simulink model "HighClearance_model"  (R2019b)
settings: configuration reference "configRef" (kept outside this file)
undefined symbols (not defined in the file): baseClearance, calSTEP1_e, calSTEP2_e, calSTEP3_e, calSTEP4_e, calTolMultiplier, errorMinSpd, heightCalibrating_e, heightDiffTolerance, heightDown_e, heightError_e, heightMovingDown_e, heightMovingUp_e, heightUnknown_e, heightUp_e, IOD_OK, IOD_Open, IOD_ScGnd, maxMedianWheelAngle, maxTransitionMachineSpd, minTransitionMachineSpd, positionSensor_tblData, positionSensorFL_BrkPnts, positionSensorFR_BrkPnts, positionSensorRL_BrkPnts, positionSensorRR_BrkPnts, step_time, trackWidthMax, trackWidthMin, trackWidthTolerance, twoWheelSteer
libraries: HighClearance_library x129, simulink x25
(part 1 of 3)
settings Model: Creator=lemaya  LastModifiedBy=lemaya
settings ConfigSetRef: SourceName=configRef  SourceLocation=Base Workspace

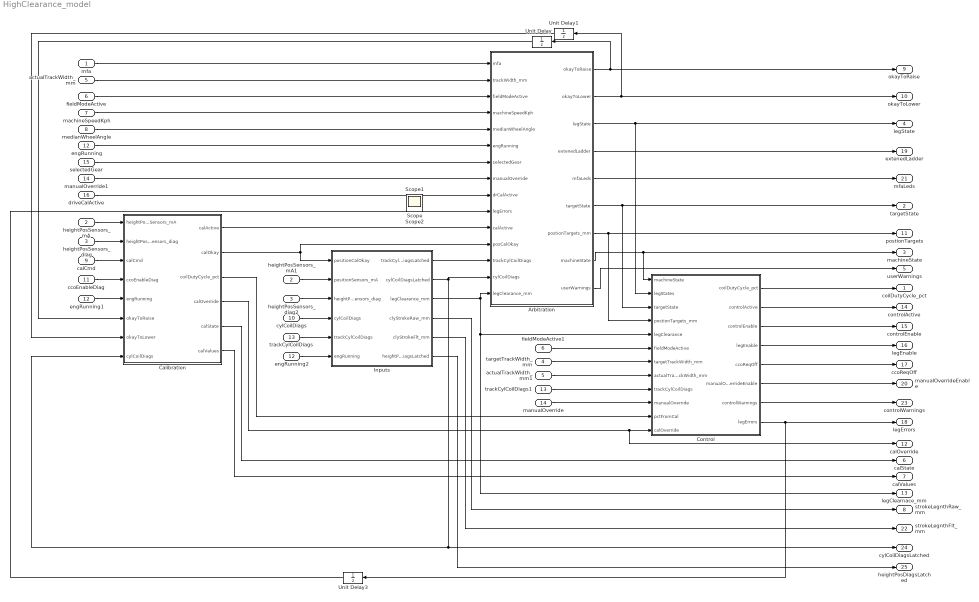
== system HighClearance_model ==
  mfa : Inport  OutDataTypeStr=Bus: MfaBus
  heightPosSensors_mA : Inport  Port=2  OutDataTypeStr=Bus: CylinderBus
  heightPosSensors_diag : Inport  Port=3  OutDataTypeStr=Bus: StateBus
  targetTrackWidth_mm : Inport  Port=4  OutDataTypeStr=Bus: CylinderBus
  actualTrackWidth_mm : Inport  Port=5  OutDataTypeStr=Bus: CylinderBus
  fieldModeActive : Inport  Port=6
  machineSpeedKph : Inport  Port=7
  medianWheelAngle : Inport  Port=8
  calCmd : Inport  Port=9
  cylCoilDiags : Inport  Port=10  OutDataTypeStr=Bus: CoilStateBus
  ccoEnableDiag : Inport  Port=11  OutDataTypeStr=uint8
  engRunning : Inport  Port=12  OutDataTypeStr=boolean
  trackCylCoilDiags : Inport  Port=13  OutDataTypeStr=Bus: CoilStateBus
  manualOverride : Inport  Port=14
  selectedGear : Inport  Port=15
  driveCalActive : Inport  Port=16
  Arbitration : Subsystem
  Calibration : Subsystem
  Control : Subsystem
  Inputs : Subsystem
  Unit Delay : UnitDelay  SampleTime=-1  HasFrameUpgradeWarning=on
  Unit Delay1 : UnitDelay  SampleTime=-1  HasFrameUpgradeWarning=on
  Unit Delay3 : UnitDelay  SampleTime=-1  HasFrameUpgradeWarning=on
  actualTrackWidth_mm1 : InportShadow  Port=5  OutDataTypeStr=Bus: CylinderBus
  engRunning1 : InportShadow  Port=12  OutDataTypeStr=boolean
  engRunning2 : InportShadow  Port=12  OutDataTypeStr=boolean
  fieldModeActive1 : InportShadow  Port=6
  heightPosSensors_diag2 : InportShadow  Port=3  OutDataTypeStr=Bus: StateBus
  heightPosSensors_mA1 : InportShadow  Port=2  OutDataTypeStr=Bus: CylinderBus
  manualOverride1 : InportShadow  Port=14
  trackCylCoilDiags1 : InportShadow  Port=13  OutDataTypeStr=Bus: CoilStateBus
  coilDutyCycle_pct : Outport  OutDataTypeStr=Bus: CoilBus
  targetState : Outport  Port=2
  machineState : Outport  Port=3
  legState : Outport  Port=4  OutDataTypeStr=Bus: StateBus
  userWarnings : Outport  Port=5  OutDataTypeStr=Bus: UserWarningBus
  calState : Outport  Port=6
  calValues : Outport  Port=7  OutDataTypeStr=Bus: CoilBus
  strokeLegnthRaw_mm : Outport  Port=8  OutDataTypeStr=Bus: CylinderBus
  okayToRaise : Outport  Port=9
  okayToLower : Outport  Port=10
  postionTargets : Outport  Port=11  OutDataTypeStr=Bus: CylinderBus
  calOverride : Outport  Port=12
  legClearnace_mm : Outport  Port=13  OutDataTypeStr=Bus: CylinderBus
  controlActive : Outport  Port=14
  controlEnable : Outport  Port=15
  legEnable : Outport  Port=16  OutDataTypeStr=Bus: StateBus
  ccoReqOff : Outport  Port=17
  legErrors : Outport  Port=18  OutDataTypeStr=Bus: ErrorsBus
  extenedLadder : Outport  Port=19
  manualOverrideEnable : Outport  Port=20
  mfaLeds : Outport  Port=21  OutDataTypeStr=Bus: MfaBus
  strokeLegnthFlt_mm : Outport  Port=22  OutDataTypeStr=Bus: CylinderBus
  controlWarnings : Outport  Port=23  OutDataTypeStr=Bus: ControlWarningsBus  BusOutputAsStruct=on
  cylCoilDiagsLatched : Outport  Port=24  OutDataTypeStr=Bus: CoilStateBus
  heightPosDiagsLatched : Outport  Port=25  OutDataTypeStr=Bus: StateBus
  Scope : Scope
  Scope1 : Scope
  Scope2 : Scope
  wires:
  heightPosSensors_mA1/1 -> Inputs/2(positionSensors_mA)
  Inputs/4(clyStrokeRaw_mm) -> strokeLegnthRaw_mm/1
  actualTrackWidth_mm/1 -> Arbitration/2(trackWidth_mm)
  mfa/1 -> Arbitration/1(mfa)
  Arbitration/7(postionTargets_mm) -> Control/4(postionTargets_mm), postionTargets/1
  actualTrackWidth_mm1/1 -> Control/8(actualTrackWidth_mm)
  Arbitration/6(targetState) -> Control/3(targetState), targetState/1
  Arbitration/8(machineState) -> Control/1(machineState), machineState/1
  Arbitration/3(legState) -> Control/2(legStates), legState/1
  fieldModeActive/1 -> Arbitration/3(fieldModeActive)
  targetTrackWidth_mm/1 -> Control/7(targetTrackWidth_mm)
  Arbitration/9(userWarnings) -> userWarnings/1
  machineSpeedKph/1 -> Arbitration/4(machineSpeedKph)
  medianWheelAngle/1 -> Arbitration/5(medianWheelAngle)
  Calibration/1(calActive) -> Arbitration/11(calActive)
  Calibration/2(calOkay) -> Inputs/1(positionCalOkay), Arbitration/12(posCalOkay)
  heightPosSensors_mA/1 -> Calibration/1(heightPosSensors_mA)
  heightPosSensors_diag/1 -> Calibration/2(heightPosSensors_diag)
  calCmd/1 -> Calibration/3(calCmd)
  Calibration/5(calState) -> calState/1
  Calibration/3(coilDutyCycle_pct) -> Control/11(pctFromCal)
  Calibration/4(calOverride) -> Control/12(calOverride), calOverride/1
  Calibration/6(calValues) -> calValues/1
  ccoEnableDiag/1 -> Calibration/4(ccoEnableDiag)
  engRunning/1 -> Arbitration/6(engRunning)
  Arbitration/1(okayToRaise) -> Unit Delay/1, okayToRaise/1
  Arbitration/2(okayToLower) -> Unit Delay1/1, okayToLower/1
  Unit Delay/1 -> Calibration/6(okayToRaise)
  Unit Delay1/1 -> Calibration/7(okayToLower)
  Control/1(coilDutyCycle_pct) -> coilDutyCycle_pct/1
  heightPosSensors_diag2/1 -> Inputs/3(heightPosSensors_diag)
  Inputs/3(legClearance_mm) -> Arbitration/15(legClearance_mm), legClearnace_mm/1, Control/5(legClearance)
  Control/2(controlActive) -> controlActive/1
  Control/3(controlEnable) -> controlEnable/1
  Control/4(legEnable) -> legEnable/1
  Control/5(ccoReqOff) -> ccoReqOff/1
  Control/8(legErrors) -> legErrors/1, Unit Delay3/1
  Unit Delay3/1 -> Arbitration/10(legErrors)
  manualOverride/1 -> Control/10(manualOverride)
  selectedGear/1 -> Arbitration/7(selectedGear)
  Arbitration/4(extenedLadder) -> extenedLadder/1
  Control/6(manualOverrideEnable) -> manualOverrideEnable/1
  Arbitration/5(mfaLeds) -> mfaLeds/1
  Inputs/5(clyStrokeFlt_mm) -> strokeLegnthFlt_mm/1
  manualOverride1/1 -> Arbitration/8(manualOverride)
  Control/7(controlWarnings) -> controlWarnings/1
  driveCalActive/1 -> Arbitration/9(drCalActive)
  cylCoilDiags/1 -> Inputs/4(cylCoilDiags)
  Inputs/2(cylCoilDiagsLatched) -> Arbitration/14(cylCoilDiags), Calibration/8(cylCoilDiags), cylCoilDiagsLatched/1
  Inputs/1(trackCylCoilDiagsLatched) -> Arbitration/13(trackCylCoilDiags)
  trackCylCoilDiags/1 -> Inputs/5(trackCylCoilDiags)
  trackCylCoilDiags1/1 -> Control/9(trackCylCoilDiags)
  engRunning1/1 -> Calibration/5(engRunning)
  fieldModeActive1/1 -> Control/6(fieldModeActive)
  Inputs/6(heightPosDiagsLatched) -> heightPosDiagsLatched/1
  engRunning2/1 -> Inputs/6(engRunning)

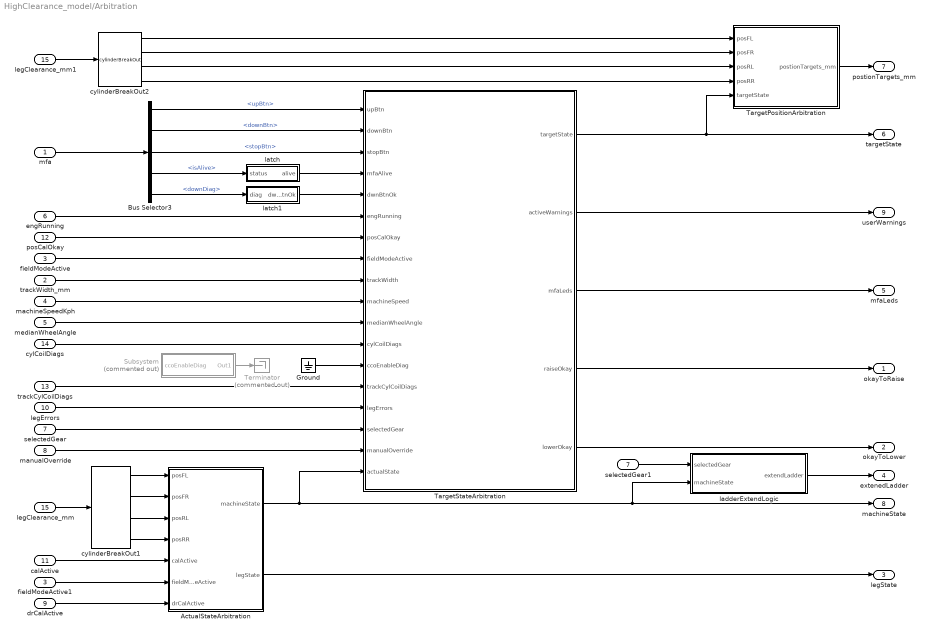
== system HighClearance_model/Arbitration ==
  mfa : Inport  OutDataTypeStr=Bus: MfaBus
  trackWidth_mm : Inport  Port=2  OutDataTypeStr=Bus: CylinderBus
  fieldModeActive : Inport  Port=3
  machineSpeedKph : Inport  Port=4
  medianWheelAngle : Inport  Port=5
  engRunning : Inport  Port=6
  selectedGear : Inport  Port=7
  manualOverride : Inport  Port=8
  drCalActive : Inport  Port=9
  legErrors : Inport  Port=10  OutDataTypeStr=Bus: ErrorsBus
  calActive : Inport  Port=11
  posCalOkay : Inport  Port=12
  trackCylCoilDiags : Inport  Port=13  OutDataTypeStr=Bus: CoilStateBus
  cylCoilDiags : Inport  Port=14  OutDataTypeStr=Bus: CoilStateBus
  legClearance_mm : Inport  Port=15  OutDataTypeStr=Bus: CylinderBus
  ActualStateArbitration : Subsystem
  Bus Selector3 : BusSelector  OutputSignals=upBtn,downBtn,stopBtn,isAlive,downDiag
  Ground : Ground
  Subsystem : Subsystem  Commented=on
  TargetPositionArbitration : Subsystem
  TargetStateArbitration : Stateflow chart  TreatAsAtomicUnit=on
  Terminator : Terminator  Commented=on
  cylinderBreakOut1 : HighClearance_library/cylinderBreakOut  SystemSampleTime=-1  Latency=0  AutoFrameSizeCalculation=off
  cylinderBreakOut2 : HighClearance_library/cylinderBreakOut  SystemSampleTime=-1  Latency=0  AutoFrameSizeCalculation=off
  fieldModeActive1 : InportShadow  Port=3
  ladderExtendLogic : Stateflow chart  TreatAsAtomicUnit=on
      settings: AttributesFormatString=%<Description> Note: Ladder extention not used
  latch : Stateflow chart  TreatAsAtomicUnit=on
  latch1 : Stateflow chart  TreatAsAtomicUnit=on
  legClearance_mm1 : InportShadow  Port=15  OutDataTypeStr=Bus: CylinderBus
  selectedGear1 : InportShadow  Port=7
  okayToRaise : Outport
  okayToLower : Outport  Port=2
  legState : Outport  Port=3  OutDataTypeStr=Bus: StateBus
  extenedLadder : Outport  Port=4
  mfaLeds : Outport  Port=5  OutDataTypeStr=Bus: MfaBus
  targetState : Outport  Port=6
  postionTargets_mm : Outport  Port=7  OutDataTypeStr=Bus: CylinderBus
  machineState : Outport  Port=8
  userWarnings : Outport  Port=9  OutDataTypeStr=Bus: UserWarningBus
  wires:
  ActualStateArbitration/2(legState) -> legState/1
  ActualStateArbitration/1(machineState) -> TargetStateArbitration/18(actualState), ladderExtendLogic/2(machineState), machineState/1
  TargetStateArbitration/1(targetState) -> targetState/1, TargetPositionArbitration/5(targetState)
  TargetPositionArbitration/1(postionTargets_mm) -> postionTargets_mm/1
  mfa/1 -> Bus Selector3/1
  Bus Selector3/2 -> TargetStateArbitration/2(downBtn)  "<downBtn>"
  Bus Selector3/1 -> TargetStateArbitration/1(upBtn)  "<upBtn>"
  Bus Selector3/3 -> TargetStateArbitration/3(stopBtn)  "<stopBtn>"
  TargetStateArbitration/2(activeWarnings) -> userWarnings/1
  calActive/1 -> ActualStateArbitration/5(calActive)
  cylinderBreakOut1/4 -> ActualStateArbitration/4(posRR)
  cylinderBreakOut1/3 -> ActualStateArbitration/3(posRL)
  cylinderBreakOut1/2 -> ActualStateArbitration/2(posFR)
  cylinderBreakOut1/1 -> ActualStateArbitration/1(posFL)
  legClearance_mm/1 -> cylinderBreakOut1/1
  legClearance_mm1/1 -> cylinderBreakOut2/1
  cylinderBreakOut2/1 -> TargetPositionArbitration/1(posFL)
  cylinderBreakOut2/2 -> TargetPositionArbitration/2(posFR)
  cylinderBreakOut2/3 -> TargetPositionArbitration/3(posRL)
  cylinderBreakOut2/4 -> TargetPositionArbitration/4(posRR)
  trackWidth_mm/1 -> TargetStateArbitration/9(trackWidth)
  fieldModeActive/1 -> TargetStateArbitration/8(fieldModeActive)
  machineSpeedKph/1 -> TargetStateArbitration/10(machineSpeed)
  medianWheelAngle/1 -> TargetStateArbitration/11(medianWheelAngle)
  cylCoilDiags/1 -> TargetStateArbitration/12(cylCoilDiags)
  posCalOkay/1 -> TargetStateArbitration/7(posCalOkay)
  engRunning/1 -> TargetStateArbitration/6(engRunning)
  trackCylCoilDiags/1 -> TargetStateArbitration/14(trackCylCoilDiags)
  TargetStateArbitration/4(raiseOkay) -> okayToRaise/1
  TargetStateArbitration/5(lowerOkay) -> okayToLower/1
  legErrors/1 -> TargetStateArbitration/15(legErrors)
  selectedGear/1 -> TargetStateArbitration/16(selectedGear)
  selectedGear1/1 -> ladderExtendLogic/1(selectedGear)
  ladderExtendLogic/1(extendLadder) -> extenedLadder/1
  TargetStateArbitration/3(mfaLeds) -> mfaLeds/1
  manualOverride/1 -> TargetStateArbitration/17(manualOverride)
  Subsystem/1(Out1) -> Terminator/1
  Ground/1 -> TargetStateArbitration/13(ccoEnableDiag)
  Bus Selector3/4 -> latch/1(status)  "<isAlive>"
  latch/1(alive) -> TargetStateArbitration/4(mfaAlive)
  fieldModeActive1/1 -> ActualStateArbitration/6(fieldModeActive)
  drCalActive/1 -> ActualStateArbitration/7(drCalActive)
  Bus Selector3/5 -> latch1/1(diag)  "<downDiag>"
  latch1/1(dwnBtnOk) -> TargetStateArbitration/5(dwnBtnOk)

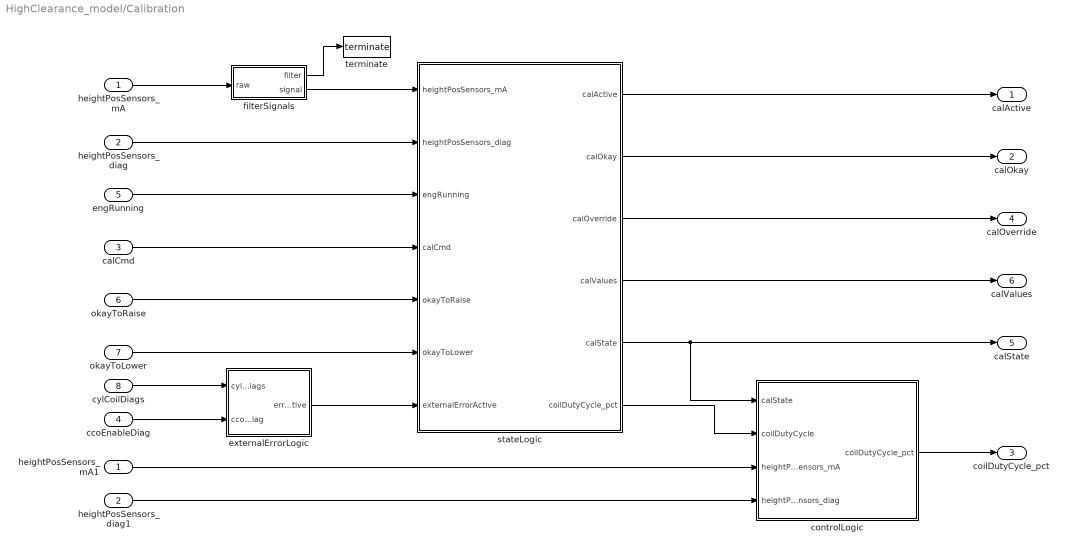
== system HighClearance_model/Calibration ==
  heightPosSensors_mA : Inport  OutDataTypeStr=Bus: CylinderBus
  heightPosSensors_diag : Inport  Port=2  OutDataTypeStr=Bus: StateBus
  calCmd : Inport  Port=3
  ccoEnableDiag : Inport  Port=4
  engRunning : Inport  Port=5  OutDataTypeStr=boolean
  okayToRaise : Inport  Port=6
  okayToLower : Inport  Port=7
  cylCoilDiags : Inport  Port=8  OutDataTypeStr=Bus: CoilStateBus
  controlLogic : Subsystem
  externalErrorLogic : Subsystem
  filterSignals : Subsystem
  heightPosSensors_diag1 : InportShadow  Port=2  OutDataTypeStr=Bus: StateBus
  heightPosSensors_mA1 : InportShadow  OutDataTypeStr=Bus: CylinderBus
  stateLogic : Subsystem
  terminate : HighClearance_library/terminate  SystemSampleTime=-1  Latency=0  AutoFrameSizeCalculation=off
  calActive : Outport
  calOkay : Outport  Port=2
  coilDutyCycle_pct : Outport  Port=3  OutDataTypeStr=Bus: CoilBus
  calOverride : Outport  Port=4
  calState : Outport  Port=5
  calValues : Outport  Port=6
  wires:
  heightPosSensors_mA/1 -> filterSignals/1(raw)
  heightPosSensors_diag/1 -> stateLogic/2(heightPosSensors_diag)
  calCmd/1 -> stateLogic/4(calCmd)
  stateLogic/1(calActive) -> calActive/1
  stateLogic/2(calOkay) -> calOkay/1
  stateLogic/5(calState) -> controlLogic/1(calState), calState/1
  stateLogic/3(calOverride) -> calOverride/1
  stateLogic/6(coilDutyCycle_pct) -> controlLogic/2(coilDutyCycle)
  heightPosSensors_mA1/1 -> controlLogic/3(heightPosSensors_mA)
  controlLogic/1(coilDutyCycle_pct) -> coilDutyCycle_pct/1
  stateLogic/4(calValues) -> calValues/1
  ccoEnableDiag/1 -> externalErrorLogic/2(ccoEnableDiag)
  cylCoilDiags/1 -> externalErrorLogic/1(cylCoilDiags)
  externalErrorLogic/1(errorActive) -> stateLogic/7(externalErrorActive)
  okayToRaise/1 -> stateLogic/5(okayToRaise)
  okayToLower/1 -> stateLogic/6(okayToLower)
  heightPosSensors_diag1/1 -> controlLogic/4(heightPosSensors_diag)
  filterSignals/1(filter) -> terminate/1
  filterSignals/2(signal) -> stateLogic/1(heightPosSensors_mA)
  engRunning/1 -> stateLogic/3(engRunning)

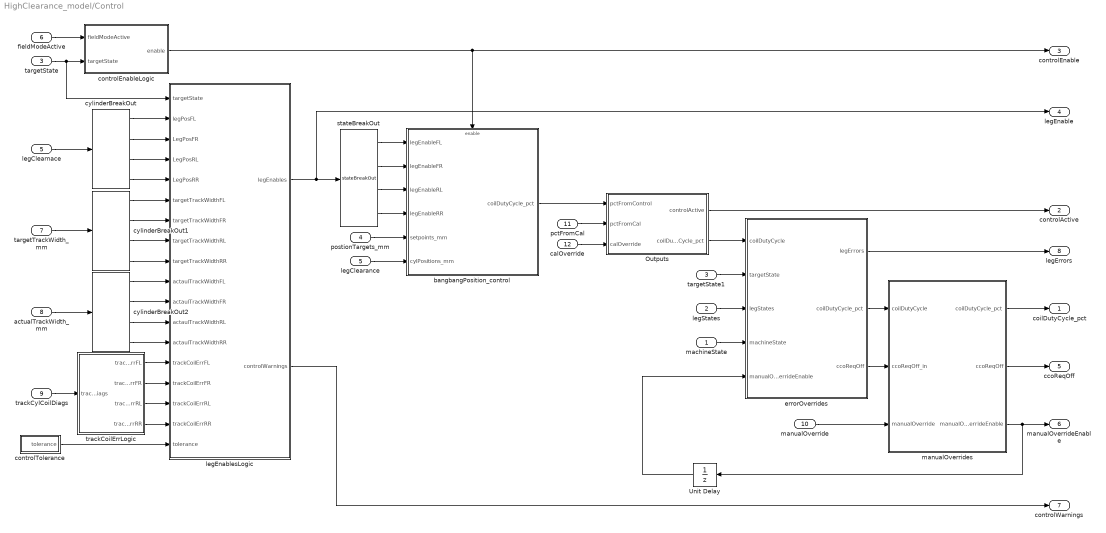
== system HighClearance_model/Control ==
  machineState : Inport
  legStates : Inport  Port=2  OutDataTypeStr=Bus: StateBus
  targetState : Inport  Port=3
  postionTargets_mm : Inport  Port=4  OutDataTypeStr=Bus: CylinderBus
  legClearance : Inport  Port=5  OutDataTypeStr=Bus: CylinderBus
  fieldModeActive : Inport  Port=6
  targetTrackWidth_mm : Inport  Port=7  OutDataTypeStr=Bus: CylinderBus
  actualTrackWidth_mm : Inport  Port=8  OutDataTypeStr=Bus: CylinderBus
  trackCylCoilDiags : Inport  Port=9  OutDataTypeStr=Bus: CoilStateBus
  manualOverride : Inport  Port=10
  pctFromCal : Inport  Port=11
  calOverride : Inport  Port=12
  Outputs : Subsystem
  Unit Delay : UnitDelay  SampleTime=-1  HasFrameUpgradeWarning=on
  bangbangPosition_control : Subsystem
  controlEnableLogic : Stateflow chart  TreatAsAtomicUnit=on
  controlTolerance : Subsystem
  cylinderBreakOut : HighClearance_library/cylinderBreakOut  SystemSampleTime=-1  Latency=0  AutoFrameSizeCalculation=off
  cylinderBreakOut1 : HighClearance_library/cylinderBreakOut  SystemSampleTime=-1  Latency=0  AutoFrameSizeCalculation=off
  cylinderBreakOut2 : HighClearance_library/cylinderBreakOut  SystemSampleTime=-1  Latency=0  AutoFrameSizeCalculation=off
  errorOverrides : Subsystem
  legClearnace : InportShadow  Port=5  OutDataTypeStr=Bus: CylinderBus
  legEnablesLogic : Subsystem
  manualOverrides : Subsystem
  stateBreakOut : HighClearance_library/stateBreakOut  SystemSampleTime=-1  Latency=0  AutoFrameSizeCalculation=off
  targetState1 : InportShadow  Port=3
  trackCoilErrLogic : Subsystem
  coilDutyCycle_pct : Outport  OutDataTypeStr=Bus: CoilBus
  controlActive : Outport  Port=2
  controlEnable : Outport  Port=3
  legEnable : Outport  Port=4
  ccoReqOff : Outport  Port=5
  manualOverrideEnable : Outport  Port=6
  controlWarnings : Outport  Port=7
  legErrors : Outport  Port=8
  wires:
  postionTargets_mm/1 -> bangbangPosition_control/5(setpoints_mm)
  legClearance/1 -> bangbangPosition_control/6(cylPositions_mm)
  controlEnableLogic/1(enable) -> bangbangPosition_control/Enable, controlEnable/1
  targetState/1 -> controlEnableLogic/2(targetState), legEnablesLogic/1(targetState)
  stateBreakOut/2 -> bangbangPosition_control/2(legEnableFR)
  stateBreakOut/3 -> bangbangPosition_control/3(legEnableRL)
  stateBreakOut/1 -> bangbangPosition_control/1(legEnableFL)
  stateBreakOut/4 -> bangbangPosition_control/4(legEnableRR)
  legEnablesLogic/1(legEnables) -> legEnable/1, stateBreakOut/1
  targetState1/1 -> errorOverrides/2(targetState)
  legStates/1 -> errorOverrides/3(legStates)
  cylinderBreakOut/1 -> legEnablesLogic/2(legPosFL)
  cylinderBreakOut/2 -> legEnablesLogic/3(LegPosFR)
  cylinderBreakOut/3 -> legEnablesLogic/4(LegPosRL)
  cylinderBreakOut/4 -> legEnablesLogic/5(LegPosRR)
  legClearnace/1 -> cylinderBreakOut/1
  cylinderBreakOut1/2 -> legEnablesLogic/7(targetTrackWidthFR)
  cylinderBreakOut1/1 -> legEnablesLogic/6(targetTrackWidthFL)
  cylinderBreakOut1/3 -> legEnablesLogic/8(targetTrackWidthRL)
  cylinderBreakOut1/4 -> legEnablesLogic/9(targetTrackWidthRR)
  targetTrackWidth_mm/1 -> cylinderBreakOut1/1
  actualTrackWidth_mm/1 -> cylinderBreakOut2/1
  cylinderBreakOut2/1 -> legEnablesLogic/10(actaulTrackWidthFL)
  cylinderBreakOut2/2 -> legEnablesLogic/11(actaulTrackWidthFR)
  cylinderBreakOut2/3 -> legEnablesLogic/12(actaulTrackWidthRL)
  cylinderBreakOut2/4 -> legEnablesLogic/13(actaulTrackWidthRR)
  bangbangPosition_control/1(coilDutyCycle_pct) -> Outputs/1(pctFromControl)
  Outputs/2(coilDutyCycle_pct) -> errorOverrides/1(coilDutyCycle)
  pctFromCal/1 -> Outputs/2(pctFromCal)
  calOverride/1 -> Outputs/3(calOverride)
  Outputs/1(controlActive) -> controlActive/1
  errorOverrides/1(legErrors) -> legErrors/1
  errorOverrides/3(ccoReqOff) -> manualOverrides/2(ccoReqOff_in)
  manualOverride/1 -> manualOverrides/3(manualOverride)
  manualOverrides/1(coilDutyCycle_pct) -> coilDutyCycle_pct/1
  manualOverrides/2(ccoReqOff) -> ccoReqOff/1
  manualOverrides/3(manualOverrideEnable) -> manualOverrideEnable/1, Unit Delay/1
  machineState/1 -> errorOverrides/4(machineState)
  Unit Delay/1 -> errorOverrides/5(manualOverrideEnable)
  controlTolerance/1(tolerance) -> legEnablesLogic/18(tolerance)
  legEnablesLogic/2(controlWarnings) -> controlWarnings/1
  errorOverrides/2(coilDutyCycle_pct) -> manualOverrides/1(coilDutyCycle)
  trackCylCoilDiags/1 -> trackCoilErrLogic/1(trackCylCoilDiags)
  trackCoilErrLogic/1(trackCoilErrFL) -> legEnablesLogic/14(trackCoilErrFL)
  trackCoilErrLogic/2(trackCoilErrFR) -> legEnablesLogic/15(trackCoilErrFR)
  trackCoilErrLogic/4(trackCoilErrRR) -> legEnablesLogic/17(trackCoilErrRR)
  trackCoilErrLogic/3(trackCoilErrRL) -> legEnablesLogic/16(trackCoilErrRL)
  fieldModeActive/1 -> controlEnableLogic/1(fieldModeActive)

== system HighClearance_model/Inputs ==
  positionCalOkay : Inport
  positionSensors_mA : Inport  Port=2  OutDataTypeStr=Bus: CylinderBus
  heightPosSensors_diag : Inport  Port=3  OutDataTypeStr=Bus: StateBus
  cylCoilDiags : Inport  Port=4  OutDataTypeStr=Bus: CoilStateBus
  trackCylCoilDiags : Inport  Port=5  OutDataTypeStr=Bus: CoilStateBus
  engRunning : Inport  Port=6  OutDataTypeStr=boolean
  clyCoilDiagsLatchLogic : Subsystem
  legPositions : Subsystem
  trackCylCoilDiagsLatchLogic : Subsystem
  trackCylCoilDiagsLatched : Outport  OutDataTypeStr=Bus: CoilStateBus
  cylCoilDiagsLatched : Outport  Port=2  OutDataTypeStr=Bus: CoilStateBus
  legClearance_mm : Outport  Port=3  OutDataTypeStr=Bus: CylinderBus
  clyStrokeRaw_mm : Outport  Port=4  OutDataTypeStr=Bus: CylinderBus
  clyStrokeFlt_mm : Outport  Port=5  OutDataTypeStr=Bus: CylinderBus
  heightPosDiagsLatched : Outport  Port=6  OutDataTypeStr=Bus: StateBus
  wires:
  positionSensors_mA/1 -> legPositions/1(positionSensors_mA)
  legPositions/2(clyPositionsRaw_mm) -> clyStrokeRaw_mm/1
  positionCalOkay/1 -> legPositions/2(posSensorCalOkay)
  heightPosSensors_diag/1 -> legPositions/3(heightPosSensors_diag)
  legPositions/1(legClearance_mm) -> legClearance_mm/1
  legPositions/3(clyPositionsFlt_mm) -> clyStrokeFlt_mm/1
  cylCoilDiags/1 -> clyCoilDiagsLatchLogic/1(cylCoilDiags)
  clyCoilDiagsLatchLogic/1(cylCoilDiagsLatched) -> cylCoilDiagsLatched/1
  trackCylCoilDiags/1 -> trackCylCoilDiagsLatchLogic/1(trackCylCoilDiags)
  trackCylCoilDiagsLatchLogic/1(trackCylCoilDiagsLatched) -> trackCylCoilDiagsLatched/1
  legPositions/4(heightPosDiagsLatched) -> heightPosDiagsLatched/1
  engRunning/1 -> legPositions/4(engRunning)

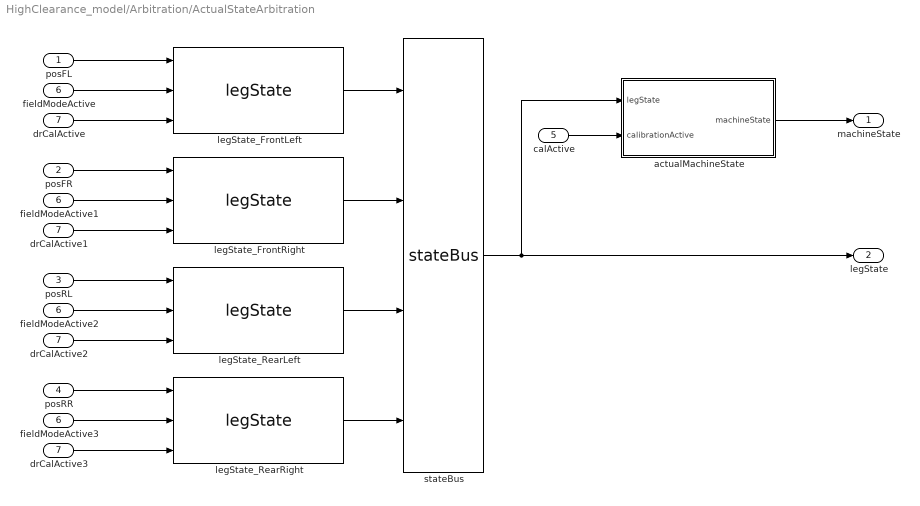
== system HighClearance_model/Arbitration/ActualStateArbitration ==
  posFL : Inport
  posFR : Inport  Port=2
  posRL : Inport  Port=3
  posRR : Inport  Port=4
  calActive : Inport  Port=5
  fieldModeActive : Inport  Port=6
  drCalActive : Inport  Port=7
  actualMachineState : Stateflow chart  TreatAsAtomicUnit=on
  drCalActive1 : InportShadow  Port=7
  drCalActive2 : InportShadow  Port=7
  drCalActive3 : InportShadow  Port=7
  fieldModeActive1 : InportShadow  Port=6
  fieldModeActive2 : InportShadow  Port=6
  fieldModeActive3 : InportShadow  Port=6
  legState_FrontLeft : HighClearance_library/legState  SystemSampleTime=-1  Latency=0  AutoFrameSizeCalculation=off
  legState_FrontRight : HighClearance_library/legState  SystemSampleTime=-1  Latency=0  AutoFrameSizeCalculation=off
  legState_RearLeft : HighClearance_library/legState  SystemSampleTime=-1  Latency=0  AutoFrameSizeCalculation=off
  legState_RearRight : HighClearance_library/legState  SystemSampleTime=-1  Latency=0  AutoFrameSizeCalculation=off
  stateBus : HighClearance_library/stateBus  SystemSampleTime=-1  Latency=0  AutoFrameSizeCalculation=off
  machineState : Outport
  legState : Outport  Port=2  OutDataTypeStr=Bus: StateBus
  wires:
  posRR/1 -> legState_RearRight/1
  posRL/1 -> legState_RearLeft/1
  posFR/1 -> legState_FrontRight/1
  posFL/1 -> legState_FrontLeft/1
  actualMachineState/1(machineState) -> machineState/1
  calActive/1 -> actualMachineState/2(calibrationActive)
  stateBus/1 -> actualMachineState/1(legState), legState/1
  legState_FrontRight/1 -> stateBus/2
  legState_FrontLeft/1 -> stateBus/1
  legState_RearRight/1 -> stateBus/4
  legState_RearLeft/1 -> stateBus/3
  fieldModeActive/1 -> legState_FrontLeft/2
  drCalActive/1 -> legState_FrontLeft/3
  fieldModeActive2/1 -> legState_RearLeft/2
  fieldModeActive1/1 -> legState_FrontRight/2
  fieldModeActive3/1 -> legState_RearRight/2
  drCalActive1/1 -> legState_FrontRight/3
  drCalActive2/1 -> legState_RearLeft/3
  drCalActive3/1 -> legState_RearRight/3

== system HighClearance_model/Arbitration/Subsystem ==
  ccoEnableDiag : Inport
  Out1 : Outport
  wires:
  ccoEnableDiag/1 -> Out1/1

== system HighClearance_model/Arbitration/TargetPositionArbitration ==
  posFL : Inport
  posFR : Inport  Port=2
  posRL : Inport  Port=3
  posRR : Inport  Port=4
  targetState : Inport  Port=5
  TargetPosition : Stateflow chart  TreatAsAtomicUnit=on
  postionTargets_mm : Outport  OutDataTypeStr=Bus: CylinderBus
  wires:
  targetState/1 -> TargetPosition/1(targetState)
  TargetPosition/1(targetPos) -> postionTargets_mm/1
  posFR/1 -> TargetPosition/3(cylPosFR)
  posRL/1 -> TargetPosition/4(cylPosRL)
  posRR/1 -> TargetPosition/5(cylPosRR)
  posFL/1 -> TargetPosition/2(cylPosFL)

== system HighClearance_model/Calibration/controlLogic ==
  calState : Inport
  coilDutyCycle : Inport  Port=2
  heightPosSensors_mA : Inport  Port=3  OutDataTypeStr=Bus: CylinderBus
  heightPosSensors_diag : Inport  Port=4  OutDataTypeStr=Bus: StateBus
  calStateConverstion : Subsystem
  cylinderBreakOut : HighClearance_library/cylinderBreakOut  SystemSampleTime=-1  Latency=0  AutoFrameSizeCalculation=off
  enableCoils : Subsystem
  grounds : HighClearance_library/grounds  SystemSampleTime=-1  Latency=0  AutoFrameSizeCalculation=off
  legEnables : Subsystem
  positionFilterLogic : HighClearance_library/positionFilterLogic  SystemSampleTime=-1  Latency=0  AutoFrameSizeCalculation=off
  postionToClearance : HighClearance_library/postionToClearance  SystemSampleTime=-1  Latency=0  AutoFrameSizeCalculation=off
  terminate : HighClearance_library/terminate  SystemSampleTime=-1  Latency=0  AutoFrameSizeCalculation=off
  terminate1 : Subsystem
  toleranceDuringCal : Subsystem
  uncalibratedPositions : HighClearance_library/uncalibratedPositions  SystemSampleTime=-1  Latency=0  AutoFrameSizeCalculation=off
  coilDutyCycle_pct : Outport  OutDataTypeStr=Bus: CoilBus
  wires:
  legEnables/1(legEnables) -> enableCoils/2(enables)
  enableCoils/1(coilDutyCycle_pct) -> coilDutyCycle_pct/1
  cylinderBreakOut/1 -> legEnables/2(legPosFL)
  cylinderBreakOut/4 -> legEnables/5(LegPosRR)
  cylinderBreakOut/2 -> legEnables/3(LegPosFR)
  cylinderBreakOut/3 -> legEnables/4(LegPosRL)
  uncalibratedPositions/1 -> positionFilterLogic/1
  coilDutyCycle/1 -> enableCoils/1(coilDutyCycle)
  heightPosSensors_mA/1 -> uncalibratedPositions/1
  calState/1 -> calStateConverstion/1(calState)
  calStateConverstion/1(targetState) -> legEnables/1(targetState)
  positionFilterLogic/2 -> postionToClearance/1
  positionFilterLogic/1 -> terminate/1
  postionToClearance/1 -> cylinderBreakOut/1
  heightPosSensors_diag/1 -> postionToClearance/3
  toleranceDuringCal/1(tolerance) -> legEnables/6(tolerance)
  postionToClearance/2 -> terminate1/1(bus)
  grounds/1 -> postionToClearance/2

== system HighClearance_model/Calibration/externalErrorLogic ==
  cylCoilDiags : Inport  OutDataTypeStr=Bus: CoilStateBus
  ccoEnableDiag : Inport  Port=2
  Compare To Constant{,1..8} (9 alike) : simulink/Logic and Bit Operations/Compare To Constant  relop=~=  const=IOD_OK  OutDataTypeStr=boolean
  Logical Operator : Logic  Operator=OR  Inputs=9  AllPortsSameDT=off  OutDataTypeStr=boolean
  coilStateBreakOut : HighClearance_library/coilStateBreakOut  SystemSampleTime=-1  Latency=0  AutoFrameSizeCalculation=off
  errorActive : Outport
  wires:
  cylCoilDiags/1 -> coilStateBreakOut/1
  coilStateBreakOut/1 -> Compare To Constant/1
  coilStateBreakOut/2 -> Compare To Constant1/1
  coilStateBreakOut/3 -> Compare To Constant2/1
  coilStateBreakOut/4 -> Compare To Constant3/1
  coilStateBreakOut/5 -> Compare To Constant4/1
  coilStateBreakOut/6 -> Compare To Constant5/1
  coilStateBreakOut/7 -> Compare To Constant6/1
  coilStateBreakOut/8 -> Compare To Constant7/1
  ccoEnableDiag/1 -> Compare To Constant8/1
  Compare To Constant/1 -> Logical Operator/1
  Compare To Constant1/1 -> Logical Operator/2
  Compare To Constant2/1 -> Logical Operator/3
  Compare To Constant3/1 -> Logical Operator/4
  Compare To Constant4/1 -> Logical Operator/5
  Compare To Constant5/1 -> Logical Operator/6
  Compare To Constant6/1 -> Logical Operator/7
  Compare To Constant7/1 -> Logical Operator/8
  Compare To Constant8/1 -> Logical Operator/9
  Logical Operator/1 -> errorActive/1

== system HighClearance_model/Calibration/filterSignals ==
  raw : Inport
  cylinderBreakOut : HighClearance_library/cylinderBreakOut  SystemSampleTime=-1  Latency=0  AutoFrameSizeCalculation=off
  cylinderBus : HighClearance_library/cylinderBus  SystemSampleTime=-1  Latency=0  AutoFrameSizeCalculation=off
  cylinderBus2 : HighClearance_library/cylinderBus  SystemSampleTime=-1  Latency=0  AutoFrameSizeCalculation=off
  filterLogicFL : HighClearance_library/filterLogic  SystemSampleTime=-1  Latency=0  AutoFrameSizeCalculation=off
  filterLogicFR : HighClearance_library/filterLogic  SystemSampleTime=-1  Latency=0  AutoFrameSizeCalculation=off
  filterLogicRL : HighClearance_library/filterLogic  SystemSampleTime=-1  Latency=0  AutoFrameSizeCalculation=off
  filterLogicRR : HighClearance_library/filterLogic  SystemSampleTime=-1  Latency=0  AutoFrameSizeCalculation=off
  filter : Outport
  signal : Outport  Port=2
  wires:
  filterLogicRR/2 -> cylinderBus2/4
  filterLogicRL/2 -> cylinderBus2/3
  filterLogicFR/2 -> cylinderBus2/2
  filterLogicFL/2 -> cylinderBus2/1
  cylinderBus2/1 -> filter/1
  filterLogicRR/1 -> cylinderBus/4
  filterLogicRL/1 -> cylinderBus/3
  filterLogicFR/1 -> cylinderBus/2
  filterLogicFL/1 -> cylinderBus/1
  cylinderBus/1 -> signal/1
  raw/1 -> cylinderBreakOut/1
  cylinderBreakOut/1 -> filterLogicFL/1
  cylinderBreakOut/2 -> filterLogicFR/1
  cylinderBreakOut/3 -> filterLogicRL/1
  cylinderBreakOut/4 -> filterLogicRR/1

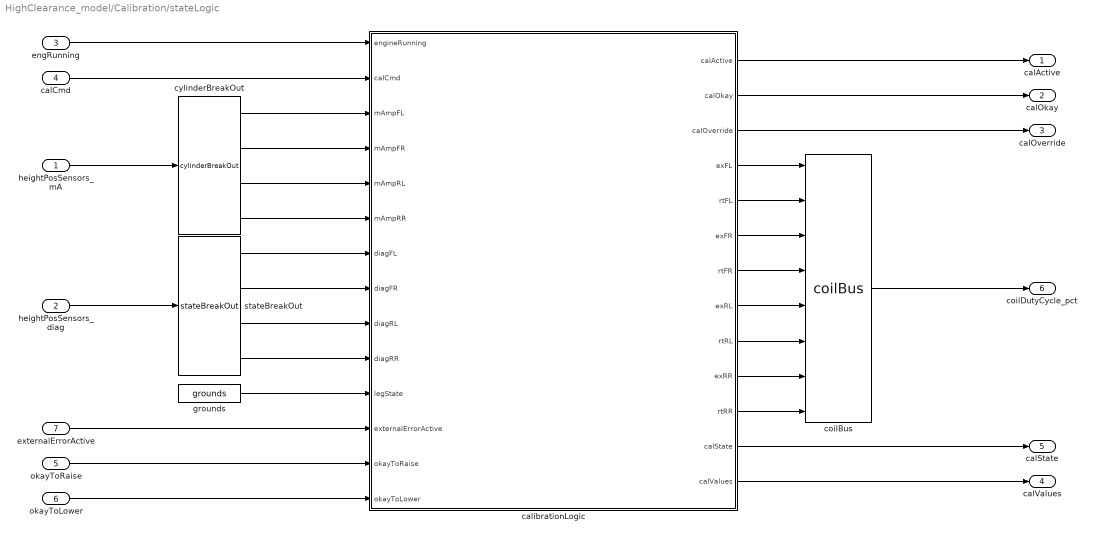
== system HighClearance_model/Calibration/stateLogic ==
  heightPosSensors_mA : Inport  OutDataTypeStr=Bus: CylinderBus
  heightPosSensors_diag : Inport  Port=2  OutDataTypeStr=Bus: StateBus
  engRunning : Inport  Port=3  OutDataTypeStr=boolean
  calCmd : Inport  Port=4
  okayToRaise : Inport  Port=5
  okayToLower : Inport  Port=6
  externalErrorActive : Inport  Port=7
  calibrationLogic : Stateflow chart  TreatAsAtomicUnit=on
  coilBus : HighClearance_library/coilBus  SystemSampleTime=-1  Latency=0  AutoFrameSizeCalculation=off
  cylinderBreakOut : HighClearance_library/cylinderBreakOut  SystemSampleTime=-1  Latency=0  AutoFrameSizeCalculation=off
  grounds : HighClearance_library/grounds  SystemSampleTime=-1  Latency=0  AutoFrameSizeCalculation=off
  stateBreakOut : HighClearance_library/stateBreakOut  SystemSampleTime=-1  Latency=0  AutoFrameSizeCalculation=off
  calActive : Outport
  calOkay : Outport  Port=2
  calOverride : Outport  Port=3
  calValues : Outport  Port=4
  calState : Outport  Port=5
  coilDutyCycle_pct : Outport  Port=6  OutDataTypeStr=Bus: CoilBus
  wires:
  heightPosSensors_mA/1 -> cylinderBreakOut/1
  coilBus/1 -> coilDutyCycle_pct/1
  calibrationLogic/3(calOverride) -> calOverride/1
  calibrationLogic/4(exFL) -> coilBus/1
  calibrationLogic/5(rtFL) -> coilBus/2
  calibrationLogic/6(exFR) -> coilBus/3
  calibrationLogic/7(rtFR) -> coilBus/4
  calibrationLogic/8(exRL) -> coilBus/5
  calibrationLogic/9(rtRL) -> coilBus/6
  calibrationLogic/10(exRR) -> coilBus/7
  calibrationLogic/11(rtRR) -> coilBus/8
  calibrationLogic/12(calState) -> calState/1
  calCmd/1 -> calibrationLogic/2(calCmd)
  calibrationLogic/1(calActive) -> calActive/1
  calibrationLogic/13(calValues) -> calValues/1
  externalErrorActive/1 -> calibrationLogic/12(externalErrorActive)
  calibrationLogic/2(calOkay) -> calOkay/1
  cylinderBreakOut/3 -> calibrationLogic/5(mAmpRL)
  cylinderBreakOut/2 -> calibrationLogic/4(mAmpFR)
  cylinderBreakOut/4 -> calibrationLogic/6(mAmpRR)
  stateBreakOut/1 -> calibrationLogic/7(diagFL)
  stateBreakOut/2 -> calibrationLogic/8(diagFR)
  stateBreakOut/3 -> calibrationLogic/9(diagRL)
  stateBreakOut/4 -> calibrationLogic/10(diagRR)
  heightPosSensors_diag/1 -> stateBreakOut/1
  okayToRaise/1 -> calibrationLogic/13(okayToRaise)
  okayToLower/1 -> calibrationLogic/14(okayToLower)
  cylinderBreakOut/1 -> calibrationLogic/3(mAmpFL)
  engRunning/1 -> calibrationLogic/1(engineRunning)
  grounds/1 -> calibrationLogic/11(legState)

== system HighClearance_model/Control/Outputs ==
  pctFromControl : Inport
  pctFromCal : Inport  Port=2
  calOverride : Inport  Port=3
  Compare To Zero{,1..7} (8 alike) : simulink/Logic and Bit Operations/Compare To Zero  relop=~=  OutDataTypeStr=boolean
  Logical Operator : Logic  Operator=OR  Inputs=8  AllPortsSameDT=off  OutDataTypeStr=boolean
  Switch : Switch  Criteria=u2 > Threshold
  coilBreakOut : HighClearance_library/coilBreakOut  SystemSampleTime=-1  Latency=0  AutoFrameSizeCalculation=off
  controlActive : Outport
  coilDutyCycle_pct : Outport  Port=2
  wires:
  pctFromCal/1 -> Switch/1
  Switch/1 -> coilBreakOut/1, coilDutyCycle_pct/1
  pctFromControl/1 -> Switch/3
  calOverride/1 -> Switch/2
  coilBreakOut/1 -> Compare To Zero/1
  coilBreakOut/3 -> Compare To Zero2/1
  coilBreakOut/2 -> Compare To Zero1/1
  coilBreakOut/4 -> Compare To Zero3/1
  coilBreakOut/5 -> Compare To Zero4/1
  coilBreakOut/6 -> Compare To Zero5/1
  coilBreakOut/7 -> Compare To Zero6/1
  coilBreakOut/8 -> Compare To Zero7/1
  Compare To Zero1/1 -> Logical Operator/2
  Compare To Zero3/1 -> Logical Operator/4
  Compare To Zero7/1 -> Logical Operator/8
  Compare To Zero6/1 -> Logical Operator/7
  Compare To Zero/1 -> Logical Operator/1
  Compare To Zero4/1 -> Logical Operator/5
  Compare To Zero2/1 -> Logical Operator/3
  Compare To Zero5/1 -> Logical Operator/6
  Logical Operator/1 -> controlActive/1

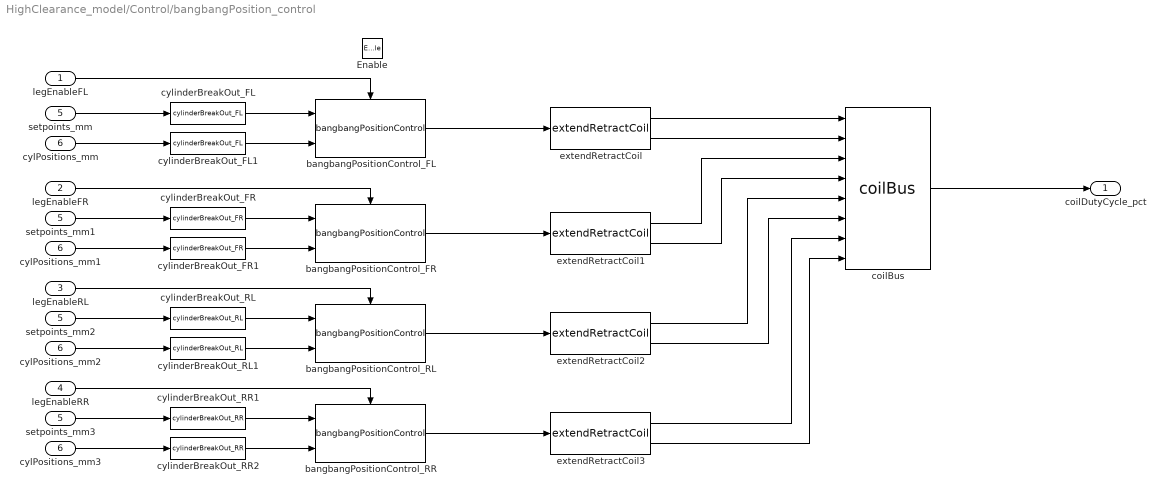
== system HighClearance_model/Control/bangbangPosition_control ==
  legEnableFL : Inport
  legEnableFR : Inport  Port=2
  legEnableRL : Inport  Port=3
  legEnableRR : Inport  Port=4
  setpoints_mm : Inport  Port=5  OutDataTypeStr=Bus: CylinderBus
  cylPositions_mm : Inport  Port=6  OutDataTypeStr=Bus: CylinderBus
  Enable : EnablePort  StatesWhenEnabling=reset
  bangbangPositionControl_FL : HighClearance_library/bangbangPositionControl  SystemSampleTime=-1  Latency=0  AutoFrameSizeCalculation=off
  bangbangPositionControl_FR : HighClearance_library/bangbangPositionControl  SystemSampleTime=-1  Latency=0  AutoFrameSizeCalculation=off
  bangbangPositionControl_RL : HighClearance_library/bangbangPositionControl  SystemSampleTime=-1  Latency=0  AutoFrameSizeCalculation=off
  bangbangPositionControl_RR : HighClearance_library/bangbangPositionControl  SystemSampleTime=-1  Latency=0  AutoFrameSizeCalculation=off
  coilBus : HighClearance_library/coilBus  SystemSampleTime=-1  Latency=0  AutoFrameSizeCalculation=off
  cylPositions_mm1 : InportShadow  Port=6  OutDataTypeStr=Bus: CylinderBus
  cylPositions_mm2 : InportShadow  Port=6  OutDataTypeStr=Bus: CylinderBus
  cylPositions_mm3 : InportShadow  Port=6  OutDataTypeStr=Bus: CylinderBus
  cylinderBreakOut_FL : HighClearance_library/cylinderBreakOut_FL  SystemSampleTime=-1  Latency=0  AutoFrameSizeCalculation=off
  cylinderBreakOut_FL1 : HighClearance_library/cylinderBreakOut_FL  SystemSampleTime=-1  Latency=0  AutoFrameSizeCalculation=off
  cylinderBreakOut_FR : HighClearance_library/cylinderBreakOut_FR  SystemSampleTime=-1  Latency=0  AutoFrameSizeCalculation=off
  cylinderBreakOut_FR1 : HighClearance_library/cylinderBreakOut_FR  SystemSampleTime=-1  Latency=0  AutoFrameSizeCalculation=off
  cylinderBreakOut_RL : HighClearance_library/cylinderBreakOut_RL  SystemSampleTime=-1  Latency=0  AutoFrameSizeCalculation=off
  cylinderBreakOut_RL1 : HighClearance_library/cylinderBreakOut_RL  SystemSampleTime=-1  Latency=0  AutoFrameSizeCalculation=off
  cylinderBreakOut_RR1 : HighClearance_library/cylinderBreakOut_RR  SystemSampleTime=-1  Latency=0  AutoFrameSizeCalculation=off
  cylinderBreakOut_RR2 : HighClearance_library/cylinderBreakOut_RR  SystemSampleTime=-1  Latency=0  AutoFrameSizeCalculation=off
  extendRetractCoil{,1..3} (4 alike) : HighClearance_library/extendRetractCoil  SystemSampleTime=-1  Latency=0  AutoFrameSizeCalculation=off
  setpoints_mm1 : InportShadow  Port=5  OutDataTypeStr=Bus: CylinderBus
  setpoints_mm2 : InportShadow  Port=5  OutDataTypeStr=Bus: CylinderBus
  setpoints_mm3 : InportShadow  Port=5  OutDataTypeStr=Bus: CylinderBus
  coilDutyCycle_pct : Outport  OutDataTypeStr=Bus: CoilBus  OutputWhenDisabled=reset  InitialOutput=[0]
  wires:
  setpoints_mm/1 -> cylinderBreakOut_FL/1
  cylPositions_mm/1 -> cylinderBreakOut_FL1/1
  cylPositions_mm2/1 -> cylinderBreakOut_RL1/1
  setpoints_mm2/1 -> cylinderBreakOut_RL/1
  setpoints_mm3/1 -> cylinderBreakOut_RR1/1
  cylPositions_mm3/1 -> cylinderBreakOut_RR2/1
  setpoints_mm1/1 -> cylinderBreakOut_FR/1
  cylPositions_mm1/1 -> cylinderBreakOut_FR1/1
  coilBus/1 -> coilDutyCycle_pct/1
  cylinderBreakOut_FL/1 -> bangbangPositionControl_FL/1
  cylinderBreakOut_FL1/1 -> bangbangPositionControl_FL/2
  bangbangPositionControl_FL/1 -> extendRetractCoil/1
  cylinderBreakOut_FR/1 -> bangbangPositionControl_FR/1
  cylinderBreakOut_FR1/1 -> bangbangPositionControl_FR/2
  cylinderBreakOut_RL1/1 -> bangbangPositionControl_RL/2
  cylinderBreakOut_RL/1 -> bangbangPositionControl_RL/1
  cylinderBreakOut_RR1/1 -> bangbangPositionControl_RR/1
  cylinderBreakOut_RR2/1 -> bangbangPositionControl_RR/2
  bangbangPositionControl_FR/1 -> extendRetractCoil1/1
  bangbangPositionControl_RL/1 -> extendRetractCoil2/1
  bangbangPositionControl_RR/1 -> extendRetractCoil3/1
  extendRetractCoil1/1 -> coilBus/3
  extendRetractCoil2/2 -> coilBus/6
  extendRetractCoil1/2 -> coilBus/4
  extendRetractCoil2/1 -> coilBus/5
  extendRetractCoil/1 -> coilBus/1
  extendRetractCoil3/2 -> coilBus/8
  extendRetractCoil/2 -> coilBus/2
  extendRetractCoil3/1 -> coilBus/7
  legEnableFL/1 -> bangbangPositionControl_FL/Enable
  legEnableFR/1 -> bangbangPositionControl_FR/Enable
  legEnableRL/1 -> bangbangPositionControl_RL/Enable
  legEnableRR/1 -> bangbangPositionControl_RR/Enable

== system HighClearance_model/Control/controlTolerance ==
  Constant : Constant  Value=heightDiffTolerance
  tolerance : Outport
  wires:
  Constant/1 -> tolerance/1

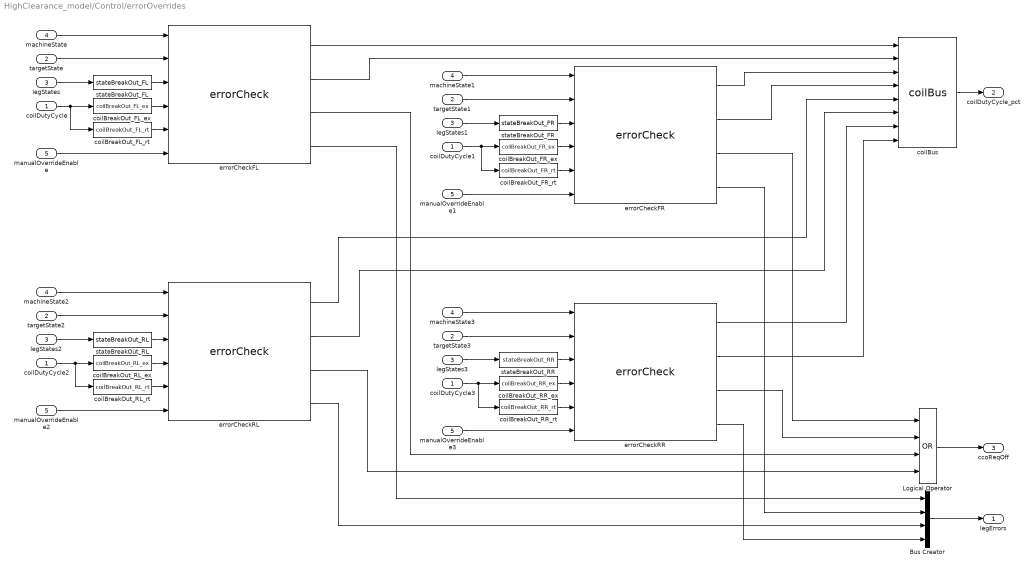
== system HighClearance_model/Control/errorOverrides ==
  coilDutyCycle : Inport
  targetState : Inport  Port=2
  legStates : Inport  Port=3  OutDataTypeStr=Bus: StateBus
  machineState : Inport  Port=4
  manualOverrideEnable : Inport  Port=5
  Bus Creator : BusCreator  Inputs=4  OutDataTypeStr=Bus: ErrorsBus
      settings: InheritFromInputs=off
  Logical Operator : Logic  Operator=OR  Inputs=4  AllPortsSameDT=off  OutDataTypeStr=boolean
  coilBreakOut_FL_ex : HighClearance_library/coilBreakOut_FL_ex  SystemSampleTime=-1  Latency=0  AutoFrameSizeCalculation=off
  coilBreakOut_FL_rt : HighClearance_library/coilBreakOut_FL_rt  SystemSampleTime=-1  Latency=0  AutoFrameSizeCalculation=off
  coilBreakOut_FR_ex : HighClearance_library/coilBreakOut_FR_ex  SystemSampleTime=-1  Latency=0  AutoFrameSizeCalculation=off
  coilBreakOut_FR_rt : HighClearance_library/coilBreakOut_FR_rt  SystemSampleTime=-1  Latency=0  AutoFrameSizeCalculation=off
  coilBreakOut_RL_ex : HighClearance_library/coilBreakOut_RL_ex  SystemSampleTime=-1  Latency=0  AutoFrameSizeCalculation=off
  coilBreakOut_RL_rt : HighClearance_library/coilBreakOut_RL_rt  SystemSampleTime=-1  Latency=0  AutoFrameSizeCalculation=off
  coilBreakOut_RR_ex : HighClearance_library/coilBreakOut_RR_ex  SystemSampleTime=-1  Latency=0  AutoFrameSizeCalculation=off
  coilBreakOut_RR_rt : HighClearance_library/coilBreakOut_RR_rt  SystemSampleTime=-1  Latency=0  AutoFrameSizeCalculation=off
  coilBus : HighClearance_library/coilBus  SystemSampleTime=-1  Latency=0  AutoFrameSizeCalculation=off
  coilDutyCycle1 : InportShadow
  coilDutyCycle2 : InportShadow
  coilDutyCycle3 : InportShadow
  errorCheckFL : HighClearance_library/errorCheck  SystemSampleTime=-1  Latency=0  AutoFrameSizeCalculation=off
  errorCheckFR : HighClearance_library/errorCheck  SystemSampleTime=-1  Latency=0  AutoFrameSizeCalculation=off
  errorCheckRL : HighClearance_library/errorCheck  SystemSampleTime=-1  Latency=0  AutoFrameSizeCalculation=off
  errorCheckRR : HighClearance_library/errorCheck  SystemSampleTime=-1  Latency=0  AutoFrameSizeCalculation=off
  legStates1 : InportShadow  Port=3  OutDataTypeStr=Bus: StateBus
  legStates2 : InportShadow  Port=3  OutDataTypeStr=Bus: StateBus
  legStates3 : InportShadow  Port=3  OutDataTypeStr=Bus: StateBus
  machineState1 : InportShadow  Port=4
  machineState2 : InportShadow  Port=4
  machineState3 : InportShadow  Port=4
  manualOverrideEnable1 : InportShadow  Port=5
  manualOverrideEnable2 : InportShadow  Port=5
  manualOverrideEnable3 : InportShadow  Port=5
  stateBreakOut_FL : HighClearance_library/stateBreakOut_FL  SystemSampleTime=-1  Latency=0  AutoFrameSizeCalculation=off
  stateBreakOut_FR : HighClearance_library/stateBreakOut_FR  SystemSampleTime=-1  Latency=0  AutoFrameSizeCalculation=off
  stateBreakOut_RL : HighClearance_library/stateBreakOut_RL  SystemSampleTime=-1  Latency=0  AutoFrameSizeCalculation=off
  stateBreakOut_RR : HighClearance_library/stateBreakOut_RR  SystemSampleTime=-1  Latency=0  AutoFrameSizeCalculation=off
  targetState1 : InportShadow  Port=2
  targetState2 : InportShadow  Port=2
  targetState3 : InportShadow  Port=2
  legErrors : Outport
  coilDutyCycle_pct : Outport  Port=2  OutDataTypeStr=Bus: CoilBus
  ccoReqOff : Outport  Port=3
  wires:
  coilDutyCycle/1 -> coilBreakOut_FL_rt/1, coilBreakOut_FL_ex/1
  legStates/1 -> stateBreakOut_FL/1
  targetState/1 -> errorCheckFL/2
  stateBreakOut_FL/1 -> errorCheckFL/3
  coilBreakOut_FL_ex/1 -> errorCheckFL/4
  coilBreakOut_FL_rt/1 -> errorCheckFL/5
  coilBus/1 -> coilDutyCycle_pct/1
  errorCheckFL/1 -> coilBus/1
  errorCheckFL/2 -> coilBus/2
  coilDutyCycle1/1 -> coilBreakOut_FR_ex/1, coilBreakOut_FR_rt/1
  legStates1/1 -> stateBreakOut_FR/1
  targetState1/1 -> errorCheckFR/2
  coilDutyCycle2/1 -> coilBreakOut_RL_rt/1, coilBreakOut_RL_ex/1
  legStates2/1 -> stateBreakOut_RL/1
  targetState2/1 -> errorCheckRL/2
  coilDutyCycle3/1 -> coilBreakOut_RR_ex/1, coilBreakOut_RR_rt/1
  legStates3/1 -> stateBreakOut_RR/1
  targetState3/1 -> errorCheckRR/2
  errorCheckFR/2 -> coilBus/4
  errorCheckFR/1 -> coilBus/3
  errorCheckRL/1 -> coilBus/5
  errorCheckRL/2 -> coilBus/6
  errorCheckRR/1 -> coilBus/7
  errorCheckRR/2 -> coilBus/8
  errorCheckRL/3 -> Logical Operator/4
  errorCheckFL/3 -> Logical Operator/3
  errorCheckRR/3 -> Logical Operator/2
  errorCheckFR/3 -> Logical Operator/1
  Logical Operator/1 -> ccoReqOff/1
  errorCheckFR/4 -> Bus Creator/2
  errorCheckRR/4 -> Bus Creator/4
  errorCheckRL/4 -> Bus Creator/3
  errorCheckFL/4 -> Bus Creator/1
  Bus Creator/1 -> legErrors/1
  machineState/1 -> errorCheckFL/1
  manualOverrideEnable/1 -> errorCheckFL/6
  machineState1/1 -> errorCheckFR/1
  machineState2/1 -> errorCheckRL/1
  machineState3/1 -> errorCheckRR/1
  coilBreakOut_FR_rt/1 -> errorCheckFR/5
  coilBreakOut_FR_ex/1 -> errorCheckFR/4
  stateBreakOut_FR/1 -> errorCheckFR/3
  manualOverrideEnable1/1 -> errorCheckFR/6
  coilBreakOut_RL_rt/1 -> errorCheckRL/5
  coilBreakOut_RL_ex/1 -> errorCheckRL/4
  stateBreakOut_RL/1 -> errorCheckRL/3
  manualOverrideEnable2/1 -> errorCheckRL/6
  coilBreakOut_RR_rt/1 -> errorCheckRR/5
  coilBreakOut_RR_ex/1 -> errorCheckRR/4
  stateBreakOut_RR/1 -> errorCheckRR/3
  manualOverrideEnable3/1 -> errorCheckRR/6

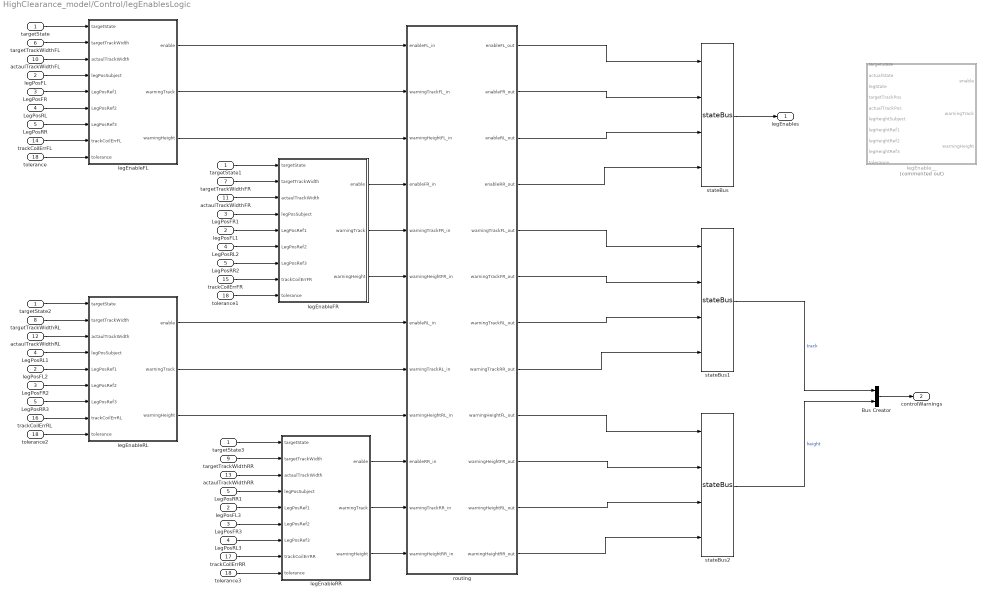
== system HighClearance_model/Control/legEnablesLogic ==
  targetState : Inport
  legPosFL : Inport  Port=2
  LegPosFR : Inport  Port=3
  LegPosRL : Inport  Port=4
  LegPosRR : Inport  Port=5
  targetTrackWidthFL : Inport  Port=6
  targetTrackWidthFR : Inport  Port=7
  targetTrackWidthRL : Inport  Port=8
  targetTrackWidthRR : Inport  Port=9
  actaulTrackWidthFL : Inport  Port=10
  actaulTrackWidthFR : Inport  Port=11
  actaulTrackWidthRL : Inport  Port=12
  actaulTrackWidthRR : Inport  Port=13
  trackCoilErrFL : Inport  Port=14
  trackCoilErrFR : Inport  Port=15
  trackCoilErrRL : Inport  Port=16
  trackCoilErrRR : Inport  Port=17
  tolerance : Inport  Port=18
  Bus Creator : BusCreator  Inputs=2  OutDataTypeStr=Bus: ControlWarningsBus  NonVirtualBus=on
  LegPosFR1 : InportShadow  Port=3
  LegPosFR2 : InportShadow  Port=3
  LegPosFR3 : InportShadow  Port=3
  LegPosRL1 : InportShadow  Port=4
  LegPosRL2 : InportShadow  Port=4
  LegPosRL3 : InportShadow  Port=4
  LegPosRR1 : InportShadow  Port=5
  LegPosRR2 : InportShadow  Port=5
  LegPosRR3 : InportShadow  Port=5
  legEnableFL : Subsystem
  legEnableFR : Subsystem
  legEnableRL : Subsystem
  legEnableRR : Subsystem
  legEnable__ : Stateflow chart  Commented=on  TreatAsAtomicUnit=on
  legPosFL1 : InportShadow  Port=2
  legPosFL2 : InportShadow  Port=2
  legPosFL3 : InportShadow  Port=2
  routing : Subsystem
  stateBus : HighClearance_library/stateBus  SystemSampleTime=-1  Latency=0  AutoFrameSizeCalculation=off
  stateBus1 : HighClearance_library/stateBus  SystemSampleTime=-1  Latency=0  AutoFrameSizeCalculation=off
  stateBus2 : HighClearance_library/stateBus  SystemSampleTime=-1  Latency=0  AutoFrameSizeCalculation=off
  targetState1 : InportShadow
  targetState2 : InportShadow
  targetState3 : InportShadow
  tolerance1 : InportShadow  Port=18
  tolerance2 : InportShadow  Port=18
  tolerance3 : InportShadow  Port=18
  legEnables : Outport
  controlWarnings : Outport  Port=2
  wires:
  stateBus/1 -> legEnables/1
  tolerance/1 -> legEnableFL/9(tolerance)
  legPosFL/1 -> legEnableFL/4(legPosSubject)
  LegPosFR/1 -> legEnableFL/5(LegPosRef1)
  LegPosRL/1 -> legEnableFL/6(LegPosRef2)
  LegPosRR/1 -> legEnableFL/7(LegPosRef3)
  actaulTrackWidthFL/1 -> legEnableFL/3(actaulTrackWidth)
  targetTrackWidthFL/1 -> legEnableFL/2(targetTrackWidth)
  targetState/1 -> legEnableFL/1(targetState)
  targetTrackWidthFR/1 -> legEnableFR/2(targetTrackWidth)
  actaulTrackWidthFR/1 -> legEnableFR/3(actaulTrackWidth)
  LegPosFR1/1 -> legEnableFR/4(legPosSubject)
  LegPosRL2/1 -> legEnableFR/6(LegPosRef2)
  LegPosRR2/1 -> legEnableFR/7(LegPosRef3)
  legPosFL1/1 -> legEnableFR/5(LegPosRef1)
  targetState1/1 -> legEnableFR/1(targetState)
  targetTrackWidthRL/1 -> legEnableRL/2(targetTrackWidth)
  actaulTrackWidthRL/1 -> legEnableRL/3(actaulTrackWidth)
  LegPosFR2/1 -> legEnableRL/6(LegPosRef2)
  LegPosRL1/1 -> legEnableRL/4(legPosSubject)
  LegPosRR3/1 -> legEnableRL/7(LegPosRef3)
  legPosFL2/1 -> legEnableRL/5(LegPosRef1)
  targetState2/1 -> legEnableRL/1(targetState)
  targetTrackWidthRR/1 -> legEnableRR/2(targetTrackWidth)
  actaulTrackWidthRR/1 -> legEnableRR/3(actaulTrackWidth)
  LegPosFR3/1 -> legEnableRR/6(LegPosRef2)
  LegPosRL3/1 -> legEnableRR/7(LegPosRef3)
  LegPosRR1/1 -> legEnableRR/4(legPosSubject)
  legPosFL3/1 -> legEnableRR/5(LegPosRef1)
  targetState3/1 -> legEnableRR/1(targetState)
  legEnableFL/1(enable) -> routing/1(enableFL_in)
  legEnableFL/2(warningTrack) -> routing/2(warningTrackFL_in)
  legEnableFL/3(warningHeight) -> routing/3(warningHeightFL_in)
  legEnableFR/1(enable) -> routing/4(enableFR_in)
  legEnableFR/2(warningTrack) -> routing/5(warningTrackFR_in)
  legEnableFR/3(warningHeight) -> routing/6(warningHeightFR_in)
  legEnableRL/1(enable) -> routing/7(enableRL_in)
  legEnableRL/2(warningTrack) -> routing/8(warningTrackRL_in)
  legEnableRL/3(warningHeight) -> routing/9(warningHeightRL_in)
  legEnableRR/1(enable) -> routing/10(enableRR_in)
  legEnableRR/2(warningTrack) -> routing/11(warningTrackRR_in)
  legEnableRR/3(warningHeight) -> routing/12(warningHeightRR_in)
  routing/1(enableFL_out) -> stateBus/1
  routing/2(enableFR_out) -> stateBus/2
  routing/3(enableRL_out) -> stateBus/3
  routing/4(enableRR_out) -> stateBus/4
  routing/5(warningTrackFL_out) -> stateBus1/1
  routing/6(warningTrackFR_out) -> stateBus1/2
  routing/7(warningTrackRL_out) -> stateBus1/3
  routing/8(warningTrackRR_out) -> stateBus1/4
  routing/9(warningHeightFL_out) -> stateBus2/1
  routing/10(warningHeightFR_out) -> stateBus2/2
  routing/11(warningHeightRL_out) -> stateBus2/3
  routing/12(warningHeightRR_out) -> stateBus2/4
  Bus Creator/1 -> controlWarnings/1
  stateBus1/1 -> Bus Creator/1  "track"
  stateBus2/1 -> Bus Creator/2  "height"
  trackCoilErrFL/1 -> legEnableFL/8(trackCoilErrFL)
  tolerance1/1 -> legEnableFR/9(tolerance)
  trackCoilErrFR/1 -> legEnableFR/8(trackCoilErrFR)
  tolerance3/1 -> legEnableRR/9(tolerance)
  trackCoilErrRR/1 -> legEnableRR/8(trackCoilErrRR)
  tolerance2/1 -> legEnableRL/9(tolerance)
  trackCoilErrRL/1 -> legEnableRL/8(trackCoilErrRL)

== system HighClearance_model/Control/manualOverrides ==
  coilDutyCycle : Inport
  ccoReqOff_in : Inport  Port=2
  manualOverride : Inport  Port=3
  Constant : Constant  Value=0  OutDataTypeStr=Inherit: Inherit via back propagation
  Switch : Switch  Criteria=u2 ~= 0
  Switch1 : Switch  Criteria=u2 ~= 0
  manualOverrides : Stateflow chart  TreatAsAtomicUnit=on
  coilDutyCycle_pct : Outport  OutDataTypeStr=Bus: CoilBus
  ccoReqOff : Outport  Port=2
  manualOverrideEnable : Outport  Port=3
  wires:
  Switch1/1 -> coilDutyCycle_pct/1
  manualOverrides/2(overrideEnabled) -> manualOverrideEnable/1, Switch/2, Switch1/2
  ccoReqOff_in/1 -> Switch/3
  Switch/1 -> ccoReqOff/1
  Constant/1 -> Switch/1
  manualOverride/1 -> manualOverrides/1(override)
  manualOverrides/1(pwm) -> Switch1/1
  coilDutyCycle/1 -> Switch1/3

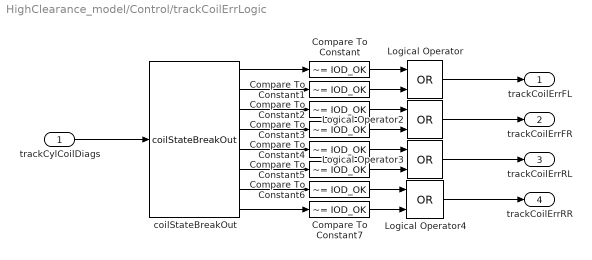
== system HighClearance_model/Control/trackCoilErrLogic ==
  trackCylCoilDiags : Inport  OutDataTypeStr=Bus: CoilStateBus
  Compare To Constant{,1..7} (8 alike) : simulink/Logic and Bit Operations/Compare To Constant  relop=~=  const=IOD_OK  OutDataTypeStr=boolean
  Logical Operator{,2..4} (4 alike) : Logic  Operator=OR  IconShape=distinctive  AllPortsSameDT=off  OutDataTypeStr=boolean
  coilStateBreakOut : HighClearance_library/coilStateBreakOut  SystemSampleTime=-1  Latency=0  AutoFrameSizeCalculation=off
  trackCoilErrFL : Outport
  trackCoilErrFR : Outport  Port=2
  trackCoilErrRL : Outport  Port=3
  trackCoilErrRR : Outport  Port=4
  wires:
  trackCylCoilDiags/1 -> coilStateBreakOut/1
  coilStateBreakOut/1 -> Compare To Constant/1
  coilStateBreakOut/2 -> Compare To Constant1/1
  coilStateBreakOut/3 -> Compare To Constant2/1
  coilStateBreakOut/4 -> Compare To Constant3/1
  coilStateBreakOut/5 -> Compare To Constant4/1
  coilStateBreakOut/6 -> Compare To Constant5/1
  coilStateBreakOut/7 -> Compare To Constant6/1
  coilStateBreakOut/8 -> Compare To Constant7/1
  Compare To Constant/1 -> Logical Operator/1
  Compare To Constant1/1 -> Logical Operator/2
  Compare To Constant3/1 -> Logical Operator2/2
  Compare To Constant2/1 -> Logical Operator2/1
  Compare To Constant5/1 -> Logical Operator3/2
  Compare To Constant4/1 -> Logical Operator3/1
  Compare To Constant7/1 -> Logical Operator4/2
  Compare To Constant6/1 -> Logical Operator4/1
  Logical Operator/1 -> trackCoilErrFL/1
  Logical Operator2/1 -> trackCoilErrFR/1
  Logical Operator3/1 -> trackCoilErrRL/1
  Logical Operator4/1 -> trackCoilErrRR/1
